simulink model "test_2DOF"  (R2024b)
settings: Solver=VariableStepAuto  StartTime=0.0  StopTime=10.0  RelTol=1e-3
libraries: cstblocks x3
settings Model: Creator=1163390615  LastModifiedBy=1163390615

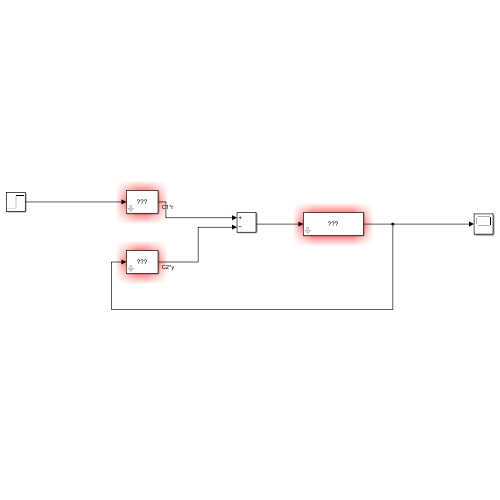
[thumbnail: Simulink's stored preview of the top-level diagram]
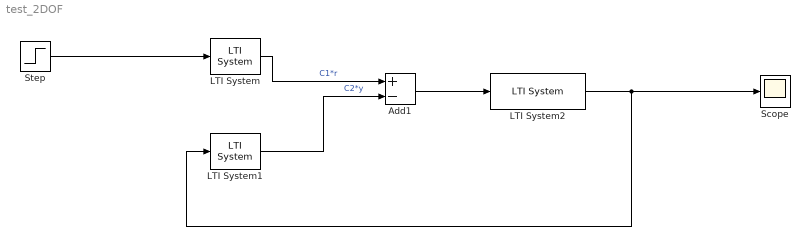
== system test_2DOF ==
  Add1 : Sum  Inputs=+-
  LTI System : cstblocks/LTI System  sys=C1  IC=[]  PadeOrder=0
  LTI System1 : cstblocks/LTI System  sys=C2  IC=[]  PadeOrder=0
  LTI System2 : cstblocks/LTI System  sys=Plant  IC=[]  PadeOrder=0
  Scope : Scope
  Step : Step  SampleTime=0
  wires:
  Step/1 -> LTI System/1
  LTI System2/1 -> LTI System1/1, Scope/1
  LTI System/1 -> Add1/1  "C1*r"
  Add1/1 -> LTI System2/1
  LTI System1/1 -> Add1/2  "C2*y"
